simulink model "error_estacionario"  (R2021a)
settings: Solver=VariableStepAuto  StartTime=0.0  StopTime=20  RelTol=1e-3
undefined symbols (not defined in the file or in its folder): i
libraries: simulink x1
settings Model: Creator=Santiago  LastModifiedBy=Santiago

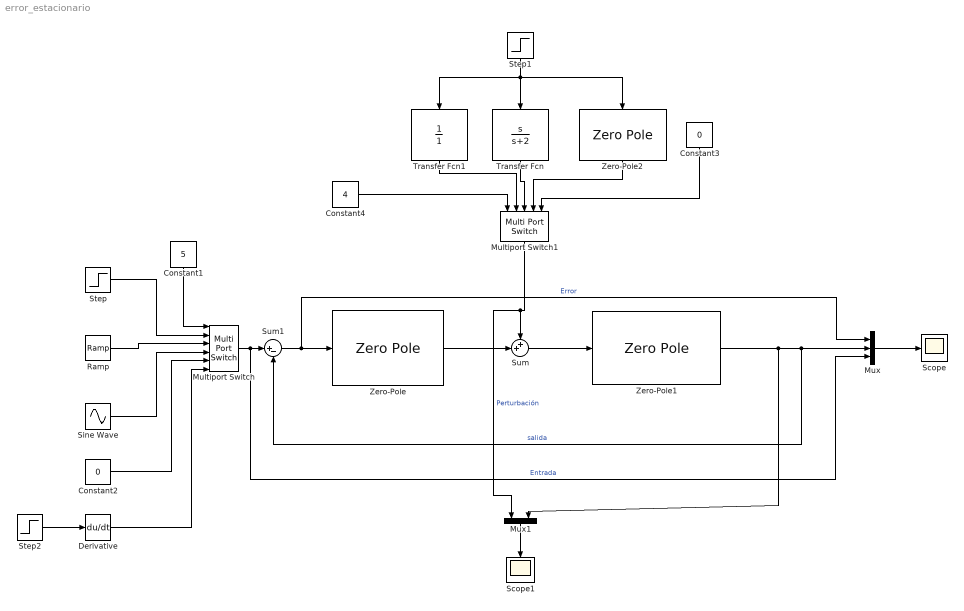
== system error_estacionario ==
  Constant1 : Constant  Value=5
  Constant2 : Constant  Value=0
  Constant3 : Constant  Value=0
  Constant4 : Constant  Value=4
  Derivative : Derivative
  Multiport Switch : MultiPortSwitch  Inputs=5
  Multiport Switch1 : MultiPortSwitch  Inputs=4
  Mux : Mux  Inputs=3
  Mux1 : Mux  Inputs=2
  Ramp : simulink/Sources/Ramp  slope=1  start=0  InitialOutput=0
  Scope : Scope
  Scope1 : Scope
  Sine Wave : Sin  SampleTime=0
  Step : Step  SampleTime=0
  Step1 : Step  SampleTime=0
  Step2 : Step  SampleTime=0
  Sum : Sum  Inputs=++|
  Sum1 : Sum  Inputs=|+-
  Transfer Fcn : TransferFcn  Numerator=[1 0]  Denominator=[1 2]
  Transfer Fcn1 : TransferFcn  Denominator=[1]
  Zero-Pole : ZeroPole  Zeros=[-8]  Poles=[-2]
  Zero-Pole1 : ZeroPole  Zeros=[-1 -1 -2]  Poles=[0 i -i -8]
  Zero-Pole2 : ZeroPole  Zeros=[0]  Poles=[-1 -1]
  wires:
  Zero-Pole1/1 -> Sum1/2, Mux/2, Mux1/2  "salida"
  Sum1/1 -> Mux/1, Zero-Pole/1  "Error"
  Zero-Pole/1 -> Sum/2
  Sum/1 -> Zero-Pole1/1
  Multiport Switch/1 -> Mux/3, Sum1/1  "Entrada"
  Constant1/1 -> Multiport Switch/1
  Step/1 -> Multiport Switch/2
  Ramp/1 -> Multiport Switch/3
  Sine Wave/1 -> Multiport Switch/4
  Mux/1 -> Scope/1
  Constant2/1 -> Multiport Switch/5
  Multiport Switch1/1 -> Mux1/1, Sum/1  "Perturbación"
  Mux1/1 -> Scope1/1
  Step1/1 -> Zero-Pole2/1, Transfer Fcn1/1, Transfer Fcn/1
  Transfer Fcn/1 -> Multiport Switch1/3
  Transfer Fcn1/1 -> Multiport Switch1/2
  Constant4/1 -> Multiport Switch1/1
  Zero-Pole2/1 -> Multiport Switch1/4
  Constant3/1 -> Multiport Switch1/5
  Step2/1 -> Derivative/1
  Derivative/1 -> Multiport Switch/6
